simulink model "linearizeB_4moments"  (R2017a)
settings: Solver=VariableStepAuto  StartTime=0.0  StopTime=10.0  RelTol=1e-3
settings Model: Creator=Luca  LastModifiedBy=Luca

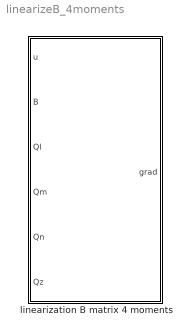
== system linearizeB_4moments ==
  linearization B matrix 4 moments : MATLAB Function  TreatAsAtomicUnit=on

== matlab function linearizeB_4moments/linearization B matrix 4 moments ==
  data: u input; B input; grad output; Ql input; Qm input; Qn input; Qz input
function grad = linearizeSystem(u, B, Ql, Qm, Qn, Qz)
%the equation here implemented comes from the article
%"A method fot including control effector interactions in the control
%allocation problem" by Oppenheimer but it is addressed to control also z
%The equation is posed in te form:

%             |u' Ql|
%             |u' Qm|
%   g = 1/2 * |u' Qn| + B
%             |u' Qz|

%and must be linearized into a new control effectiveness matrix



%check the magnitude of numbers inside the matrices
%     oom = [min(floor(log10(u+1))), min(min(floor(log10(Ql+1)))),...
%         min(min(floor(log10(Qm+1)))), min(min(floor(log10(Qn+1)))),...
%         min(min(floor(log10(Qz+1))))];
%     oom = min(oom);

oom = -1;
 
%compute the gradient that will be the new B matrix
    grad = zeros(size(B,1),length(u));
    
    ddelta = 10^(oom-5); %three orders of magnitude less than the values in the matrices
    for i = 1:length(u)
        u_base = u;
        u_incr = u; u_incr(i) = u_incr(i)+ddelta;
        u_decr = u; u_decr(i) = u_decr(i)-ddelta;
        
        g_base = ((1/2)*([u_base.'*Ql; u_base.'*Qm; u_base.'*Qn; u_base.'*Qz])+B)*u_base;
        g_incr = ((1/2)*([u_incr.'*Ql; u_incr.'*Qm; u_incr.'*Qn; u_incr.'*Qz])+B)*u_incr;
        g_decr = ((1/2)*([u_decr.'*Ql; u_decr.'*Qm; u_decr.'*Qn; u_decr.'*Qz])+B)*u_decr;
        
        grad_incr = (g_incr - g_base)/ddelta;
        grad_decr = (g_decr - g_base)/(-ddelta); 
        grad(:,i) = (grad_incr+grad_decr)/2;
    end
end
